simulink model "RetroEstadosRuidoGraficas"  (R2015a)
settings: Solver=ode45  SolverMode=SingleTasking  StartTime=0.0  StopTime=20.0  RelTol=1e-3
values from neighbouring files (symbols this model uses):
  Am = [ ... (first row only)    [Parametros.m]    (also in ParametrosOORD.m)
  amplitud = 0.1    [Parametros.m]
  Bm = [ ... (first row only)    [Parametros.m]    (also in ParametrosOORD.m)
  CIm = [0,10*pi/180,-5*pi/180,15*pi/180,0,0,0,0]'    [Parametros.m]    (also in ParametrosOORD.m = [0,0,0,0,0,0,0,0]')
  Cm = eye(8)    [Parametros.m]    (also in ParametrosOORD.m)
  Dm = zeros(8,4)    [Parametros.m]    (also in ParametrosOORD.m)
  g = 9.78    [Parametros.m]    (also in ParametrosOORD.m)
  k = 7.7e-7    (= 7.7e-07)    [Parametros.m]    (also in ParametrosOORD.m)
  m = 0.4625    [Parametros.m]    (also in ParametrosOORD.m = 0.4419)
  R = Un+K*Xn    [Parametros.m]    (also in ParametrosOORD.m = K*X+U)
  Ts = 0.02    [Parametros.m]    (also in ParametrosOORD.m)
  U = [omegaeq,omegaeq,omegaeq,omegaeq]'    [Parametros.m]    (also in ParametrosOORD.m)
  X = [zeq,0,0,0,0,0,0,0]'    [Parametros.m]    (also in ParametrosOORD.m)
  zeq = 1    [Parametros.m]    (also in ParametrosOORD.m)
undefined symbols (not defined in the file or in its folder): K
settings Model: Creator=Control  LastModifiedBy=Wally
settings DataIOCC: SignalLoggingSaveFormat=ModelDataLogs
settings OptimizationCC: BlockReduction=off  BooleanDataType=off
settings DebuggingCC: SaveWithParameterizedLinksMsg=none  UnderspecifiedInitializationDetection=Classic  MergeDetectMultiDrivingBlocksExec=none  SignalResolutionControl=TryResolveAllWithWarning  MultiTaskDSMMsg=warning  MultiTaskCondExecSysMsg=none  StateNameClashWarn=warning
settings HardwareCC: TargetUnknown=on

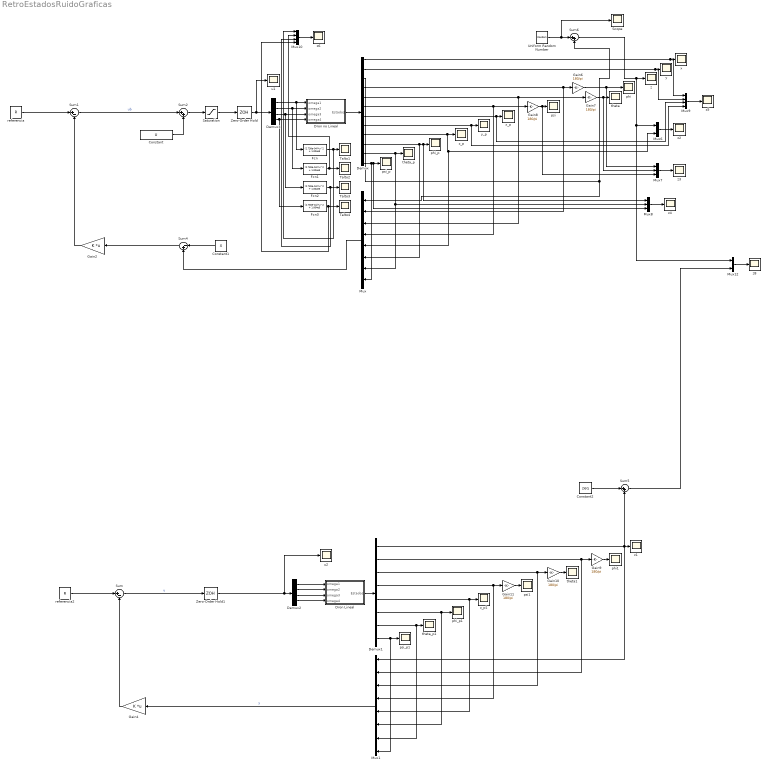
== system RetroEstadosRuidoGraficas ==
  Constant : Constant  Value=U
  Constant1 : Constant  Value=X
  Constant2 : Constant  Value=zeq
  Demux : Demux  Outputs=12
  Demux1 : Demux  Outputs=8
  Demux2 : Demux
  Demux3 : Demux
  Dron Lineal : Subsystem
  Dron no Lineal : Subsystem
  Fcn{,1..3} (4 alike) : Fcn  Expr=(2.730e-04)*u^2 + 1.004e3
  Gain{6..11} (6 alike) : Gain  Gain=180/pi
  Gain2 : Gain  Gain=K  Multiplication=Matrix(K*u) (u vector)
  Gain4 : Gain  Gain=K  Multiplication=Matrix(K*u)
  Mux : Mux  Inputs=8
  Mux1 : Mux  Inputs=8
  Mux10 : Mux
  Mux12 : Mux  Inputs=2
  Mux6 : Mux  Inputs=2
  Mux7 : Mux  Inputs=3
  Mux8 : Mux  Inputs=3
  Mux9 : Mux
  Saturation : Saturate  UpperLimit=1700  LowerLimit=1100
  Scope : Scope
      settings: SaveName=ScopeData28
  Sum : Sum  Inputs=|+-
  Sum1 : Sum  Inputs=|+-
  Sum2 : Sum  Inputs=|++
  Sum4 : Sum  Inputs=|-+
  Sum5 : Sum  Inputs=|++
  Sum6 : Sum  Inputs=|++
  Talto{1..4} (4 alike) : Scope
      Talto1 settings: SaveName=ScopeData18
      Talto2 settings: SaveName=ScopeData24
      Talto3 settings: SaveName=ScopeData25
      Talto4 settings: SaveName=ScopeData26
  Uniform Random Number : UniformRandomNumber  Minimum=-amplitud  Maximum=amplitud  SampleTime=Ts
  Zero-Order Hold : ZeroOrderHold  SampleTime=Ts
  Zero-Order Hold1 : ZeroOrderHold  SampleTime=Ts
  phi : Scope
      settings: SaveName=ScopeData3
  phi1 : Scope
      settings: SaveName=ScopeData12
  phi_p : Scope
      settings: SaveName=ScopeData9
  phi_p1 : Scope
      settings: SaveName=ScopeData13
  psi : Scope
      settings: SaveName=ScopeData5
  psi1 : Scope
      settings: SaveName=ScopeData14
  psi_p : Scope
      settings: SaveName=ScopeData11
  psi_p1 : Scope
      settings: SaveName=ScopeData15
  referencia : Constant  Value=R
  referencia2 : Constant  Value=R
  theta : Scope
      settings: SaveName=ScopeData4
  theta1 : Scope
      settings: SaveName=ScopeData16
  theta_p : Scope
      settings: SaveName=ScopeData10
  theta_p1 : Scope
      settings: SaveName=ScopeData17
  u1 : Scope
      settings: YMin=-6100  YMax=-6015  SaveName=Omega
  u2 : Scope
      settings: SaveName=ScopeData19
  x : Scope
  x_p : Scope
      settings: SaveName=ScopeData6
  y : Scope
  y_p : Scope
      settings: SaveName=ScopeData7
  z{,1..6,8} (8 alike) : Scope
      z settings: SaveName=ScopeData2
      z1 settings: TimeRange=10  SaveName=ScopeData22
      z2 settings: SaveName=Estados_z
      z3 settings: SaveName=Angulos
      z4 settings: SaveName=VelAng
      z5 settings: SaveName=XY_CI
      z6 settings: SaveName=Talto
      z8 settings: SaveName=Z_L_NL
  z_p : Scope
      settings: SaveName=ScopeData8
  z_p1 : Scope
      settings: SaveName=ScopeData23
  wires:
  Dron no Lineal/1(Estados) -> Demux/1
  Demux/1 -> Mux9/1, x/1
  Demux/2 -> Mux9/2, y/1
  Demux/5 -> Gain7/1, Mux/3
  Demux/7 -> Mux9/3, x_p/1
  Demux/8 -> Mux9/4, y_p/1
  Demux/10 -> Mux/6, Mux8/1, phi_p/1
  Dron Lineal/1(Estados) -> Demux1/1
  Demux1/1 -> Sum5/2, z1/1, Mux1/1
  Demux1/2 -> Gain9/1, Mux1/2
  Demux1/3 -> Gain10/1, Mux1/3
  Demux1/4 -> Gain11/1, Mux1/4
  Demux1/6 -> Mux1/6, phi_p1/1
  Demux1/7 -> Mux1/7, theta_p1/1
  Demux1/8 -> Mux1/8, psi_p1/1
  Demux2/1 -> Dron Lineal/1(omega1)
  Demux2/2 -> Dron Lineal/2(omega2)
  Demux2/3 -> Dron Lineal/3(omega3)
  Demux2/4 -> Dron Lineal/4(omega4)
  Sum/1 -> Zero-Order Hold1/1  "u"
  Sum1/1 -> Sum2/1  "ub"
  Constant/1 -> Sum2/2
  Demux3/1 -> Dron no Lineal/1(omega1), Fcn/1
  Demux3/2 -> Dron no Lineal/2(omega2), Fcn1/1
  Demux3/3 -> Dron no Lineal/3(omega3), Fcn2/1
  Demux3/4 -> Dron no Lineal/4(omega4), Fcn3/1
  Gain2/1 -> Sum1/2
  referencia2/1 -> Sum/1
  referencia/1 -> Sum1/1
  Sum2/1 -> Saturation/1
  Saturation/1 -> Zero-Order Hold/1
  Fcn/1 -> Mux10/1, Talto1/1
  Fcn1/1 -> Talto2/1, Mux10/2
  Fcn2/1 -> Mux10/3, Talto3/1
  Fcn3/1 -> Mux10/4, Talto4/1
  Demux/3 -> Sum6/2, Mux/1
  Demux/6 -> Gain8/1, Mux/4
  Demux/9 -> z_p/1, Mux/5, Mux6/2
  Gain4/1 -> Sum/2
  Demux1/5 -> Mux1/5, z_p1/1
  Demux/12 -> Mux/8, psi_p/1, Mux8/3
  Demux/4 -> Gain6/1, Mux/2
  Gain6/1 -> Mux7/1, phi/1
  Gain7/1 -> Mux7/2, theta/1
  Gain8/1 -> Mux7/3, psi/1
  Gain9/1 -> phi1/1
  Gain10/1 -> theta1/1
  Gain11/1 -> psi1/1
  Zero-Order Hold/1 -> Demux3/1, u1/1
  Zero-Order Hold1/1 -> u2/1, Demux2/1
  Mux6/1 -> z2/1
  Mux7/1 -> z3/1
  Mux8/1 -> z4/1
  Demux/11 -> theta_p/1, Mux/7, Mux8/2
  Mux9/1 -> z5/1
  Mux10/1 -> z6/1
  Mux12/1 -> z8/1
  Constant1/1 -> Sum4/1
  Mux/1 -> Sum4/2
  Sum4/1 -> Gain2/1
  Constant2/1 -> Sum5/1
  Sum5/1 -> Mux12/2
  Mux1/1 -> Gain4/1  "y"
  Uniform Random Number/1 -> Scope/1, Sum6/1
  Sum6/1 -> Mux12/1, Mux6/1, z/1

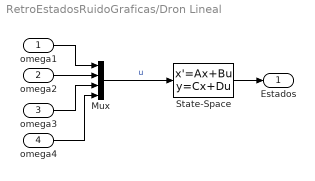
== system RetroEstadosRuidoGraficas/Dron Lineal ==
  omega1 : Inport
  omega2 : Inport  Port=2
  omega3 : Inport  Port=3
  omega4 : Inport  Port=4
  Mux : Mux
  State-Space : StateSpace  A=Am  B=Bm  C=Cm  D=Dm  X0=CIm-X
  Estados : Outport
  wires:
  omega4/1 -> Mux/4
  omega3/1 -> Mux/3
  omega2/1 -> Mux/2
  omega1/1 -> Mux/1
  State-Space/1 -> Estados/1
  Mux/1 -> State-Space/1  "u"

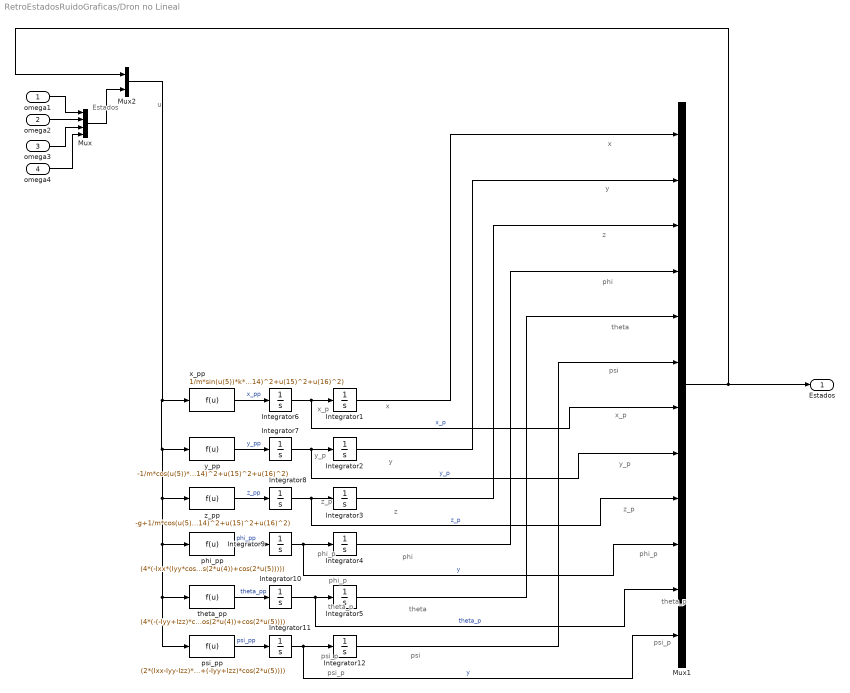
== system RetroEstadosRuidoGraficas/Dron no Lineal ==
  note: z
  note: psi_p
  note: theta_p
  note: phi_p
  note: z_p
  note: y_p
  note: x_p
  note: psi
  note: theta
  note: phi
  note: z
  note: y
  note: x
  note: psi
  note: theta
  note: phi
  note: y
  note: x
  note: psi_p
  note: theta_p
  note: phi_p
  note: z_p
  note: y_p
  note: x_p
  note: psi_p
  note: phi_p
  note: u
  note: Estados
  omega1 : Inport
  omega2 : Inport  Port=2
  omega3 : Inport  Port=3
  omega4 : Inport  Port=4
  Integrator{1..2,6..7} (4 alike) : Integrator
  Integrator10 : Integrator  InitialCondition=CIm(7)
  Integrator11 : Integrator  InitialCondition=CIm(8)
  Integrator12 : Integrator  InitialCondition=CIm(4)
  Integrator3 : Integrator  InitialCondition=CIm(1)
  Integrator4 : Integrator  InitialCondition=CIm(2)
  Integrator5 : Integrator  InitialCondition=CIm(3)
  Integrator8 : Integrator  InitialCondition=CIm(5)
  Integrator9 : Integrator  InitialCondition=CIm(6)
  Mux : Mux
  Mux1 : Mux  Inputs=12
  Mux2 : Mux  Inputs=2
  phi_pp : Fcn  Expr=(4*(-Ixx*(Iyy*cos(u(4))^2+Izz*sin(u(4))^2)*sin(u(5))*(-(Iyy-Izz)*cos(u(4))*sin(u(4))*sin(u(5))*u(11)^2+(Iyy-Izz)*cos(u(5))^2*sin(2*u(4))*u(10)*u(12)-u(11)*((Ixx+(-Iyy+Izz)*cos(2*u(4)))*cos(u(5))*u(10)+(-Ixx+Izz*cos(u(4))^2+Iyy*sin(u(4))^2)*sin(2*u(5))*u(12))+b*u(13)^2-b*u(14)^2+b*u(15)^2-b*u(16)^2)-Ixx*(Iyy-Izz)*cos(u(4))*cos(u(5))*sin(u(4))*sin(u(5))*((Iyy-Izz)*cos(u(4))*sin(u(4))*u(10)*u(11)+1/4*(2*Ixx-Iyy-Izz+(Iyy-Izz)*cos(2*u(4)))*sin(2*u(5))*u(12)^2-u(10)*(-(Iyy-Izz)*cos(u(4))*sin(u(4))*u(11)+(Ixx+(Iyy-Izz)*cos(2*u(4)))*cos(u(5))*u(12))+d*k*(u(13)^2+u(14)^2-u(15)^2-u(16)^2))-1/4*((-(Iyy+Izz)^2+(Iyy-Izz)^2*cos(4*u(4)))*cos(u(5))^2-Ixx*(4*Izz*sin(u(4))^4+Iyy*sin(2*u(4))^2))*((Ixx+(Iyy-Izz)*cos(2*u(4)))*cos(u(5))*u(11)*u(12)-1/4*(Iyy-Izz)*sin(2*u(4))*(2*u(11)^2-u(12)^2-cos(2*u(5))*u(12)^2)+d*k*(-u(13)^2+u(14)^2+u(15)^2-u(16)^2))))/(Ixx*(-(-(Iyy+Izz)^2+(Iyy-Izz)^2*cos(4*u(4)))*cos(u(5))^2+Ixx*(Iyy+Izz+(Iyy-Izz)*cos(2*u(4)))*(-cos(2*u(4))+cos(2*u(5)))))
  psi_pp : Fcn  Expr=(2*(Ixx-Iyy-Izz)*(Iyy-Izz)*cos(u(5))^2*sin(2*u(4))*u(12)*(-u(10)+sin(u(5))*u(12))-2*cos(u(5))*((-(Iyy-Izz)^2+Ixx*(Iyy+Izz))*u(10)*u(11)+(Ixx-Iyy-Izz)*(Iyy-Izz)*cos(2*u(4))*u(10)*u(11)-d*(Iyy-Izz)*k*sin(2*u(4))*(u(13)^2+u(14)^2-u(15)^2-u(16)^2))-(Iyy+Izz+(Iyy-Izz)*cos(2*u(4)))*(-(Ixx-Iyy-Izz)*sin(2*u(5))*u(11)*u(12)-2*(b*(u(13)^2-u(14)^2+u(15)^2-u(16)^2)+d*k*sin(u(5))*(u(13)^2-u(14)^2-u(15)^2+u(16)^2))))/(Ixx*(Iyy-Izz)*cos(2*u(4))^2+(-(Iyy+Izz)^2+(Iyy-Izz)^2*cos(4*u(4)))*cos(u(5))^2-Ixx*(Iyy+Izz)*cos(2*u(5))+Ixx*cos(2*u(4))*(Iyy+Izz+(-Iyy+Izz)*cos(2*u(5))))
  theta_pp : Fcn  Expr=(4*(-(-Iyy+Izz)*cos(u(4))*cos(u(5))*sin(u(4))*((Iyy-Izz)*cos(u(4))*sin(u(4))*sin(u(5))*u(11)^2-(Iyy-Izz)*cos(u(5))^2*sin(2*u(4))*u(10)*u(12)+u(11)*((Ixx+(-Iyy+Izz)*cos(2*u(4)))*cos(u(5))*u(10)+(-Ixx+Izz*cos(u(4))^2+Iyy*sin(u(4))^2)*sin(2*u(5))*u(12))-b*u(13)^2+b*u(14)^2-b*u(15)^2+b*u(16)^2)+(Izz*cos(u(4))^2*cos(u(5))^2+(Ixx+Iyy*cos(u(5))^2)*sin(u(4))^2-Ixx*sin(u(5))^2)*((Iyy-Izz)*cos(u(4))*sin(u(4))*u(10)*u(11)+1/4*(2*Ixx-Iyy-Izz+(Iyy-Izz)*cos(2*u(4)))*sin(2*u(5))*u(12)^2-u(10)*(-(Iyy-Izz)*cos(u(4))*sin(u(4))*u(11)+(Ixx+(Iyy-Izz)*cos(2*u(4)))*cos(u(5))*u(12))+d*k*(u(13)^2+u(14)^2-u(15)^2-u(16)^2))-(-Iyy+Izz)*cos(u(4))*cos(u(5))*sin(u(4))*sin(u(5))*(-(Iyy-Izz)*cos(u(4))*sin(u(4))*u(11)^2+(Ixx+(Iyy-Izz)*cos(2*u(4)))*cos(u(5))*u(11)*u(12)+(Iyy-Izz)*cos(u(4))*cos(u(5))^2*sin(u(4))*u(12)^2+d*k*(-u(13)^2+u(14)^2+u(15)^2-u(16)^2))))/(-(-(Iyy+Izz)^2+(Iyy-Izz)^2*cos(4*u(4)))*cos(u(5))^2+Ixx*(Iyy+Izz+(Iyy-Izz)*cos(2*u(4)))*(-cos(2*u(4))+cos(2*u(5))))
  x_pp : Fcn  Expr=1/m*sin(u(5))*k*(u(13)^2+u(14)^2+u(15)^2+u(16)^2)
  y_pp : Fcn  Expr=-1/m*cos(u(5))*sin(u(4))*k*(u(13)^2+u(14)^2+u(15)^2+u(16)^2)
  z_pp : Fcn  Expr=-g+1/m*cos(u(5))*cos(u(4))*k*(u(13)^2+u(14)^2+u(15)^2+u(16)^2)
  Estados : Outport
  wires:
  Mux1/1 -> Mux2/1, Estados/1
  omega1/1 -> Mux/1
  omega2/1 -> Mux/2
  omega3/1 -> Mux/3
  omega4/1 -> Mux/4
  x_pp/1 -> Integrator6/1  "x_pp"
  y_pp/1 -> Integrator7/1  "y_pp"
  z_pp/1 -> Integrator8/1  "z_pp"
  phi_pp/1 -> Integrator9/1  "phi_pp"
  theta_pp/1 -> Integrator10/1  "theta_pp"
  psi_pp/1 -> Integrator11/1  "psi_pp"
  Mux/1 -> Mux2/2
  Mux2/1 -> psi_pp/1, theta_pp/1, phi_pp/1, z_pp/1, y_pp/1, x_pp/1
  Integrator6/1 -> Mux1/7, Integrator1/1  "x_p"
  Integrator7/1 -> Mux1/8, Integrator2/1  "y_p"
  Integrator8/1 -> Mux1/9, Integrator3/1  "z_p"
  Integrator9/1 -> Integrator4/1, Mux1/10  "y"
  Integrator10/1 -> Mux1/11, Integrator5/1  "theta_p"
  Integrator11/1 -> Integrator12/1, Mux1/12  "y"
  Integrator1/1 -> Mux1/1
  Integrator2/1 -> Mux1/2
  Integrator3/1 -> Mux1/3
  Integrator4/1 -> Mux1/4
  Integrator5/1 -> Mux1/5
  Integrator12/1 -> Mux1/6
